simulink model "HMC"  (R2026a)
settings: Solver=ode1  StopTime=inf  FixedStep=0.0001
PreLoadFcn:
  | %load('C:\Users\bme_master\Desktop\mot\mot_6_deneme.mat')
  | 
  | 
  | %load('C:\Users\bme_master\Desktop\mot\PRE_G''s.mat')
PostLoadFcn:
  | , if any(exist('dsrtsu_mdlpostloadfcn', 'file') ~= 0), dsrtsu_mdlpostloadfcn('Execute', bdroot); end,
InitFcn:
  | %motor_control_init_m
  | %clear all
  | %close all
  | %clc
  | b=1e-8
  | StepSize = 1e-4;
  | N=1e-17;
  | 
  | VLV_0 =0;%120; %120
  | VA_0 = 0;%300; %300
  | VRV_0 = 0;%130;
  | VP_0 = 0;%500;
  | VLA_0 = 0;%20;
  | VV_0=5000;
  | VRA_0=0;
  | 
  | 
  | QLV_0 = 0;
  | QLA_0 = 0;
  | QP_0 = 0;
  | 
  | bh = 0;
  | th =0;
  | 
  | X_0 = [VLV_0 VA_0 VV_0 VP_0  VLA_0  VRA_0 VRV_0];
  | 
  | 
  | V0 = 10;
  | 
  | K1=.0004;%0.0001
  | K2=0.0009;%0.0009
  | KA=1;%1
  | C1=0.000000003;%0.0000003
  | lambda=6000;%3000
  | X_00 = [VLV_0 VA_0 VV_0 VRV_0];
  | 
  | r2 = 0.05/2;
  | A2 = pi*r2^2;
  | h2 = 0.63;
  | V2 = A2*h2;
  | 
  | 
  | r3 = 0.05/2;
  | A3 = pi*r3^2;
  | h3 = 0.63;
  | V3 = A3*h3;
  | 
  | 
  | rho = 997;
  | gg = 9.81;
  | %
  | init_min=0;
  | init_max=0;
  | %
  | PWM_Period =  StepSize;
  | PWM_Period_g1 = PWM_Period;
  | PWM_Period_g2 =PWM_Period;
  | PWM_Period_g3 = PWM_Period;
  | PWM_Period_g4 = PWM_Period;
  | PWM_Period_g5 = PWM_Period;
  | ... (+158 lines)
undefined symbols (not defined in the file or in its folder): Continuous, DiscIntNeverNeededParam, Time
libraries: powerlib_meascontrol x19, simulink x15, rti1202lib_adc_class1 x11, cstblocks x10, rti1202lib_dio_class1 x8, dspstat3 x3, rti1202lib_dac_class1 x1, dspswit3 x1, ctrlSharedLib x1, slpidlib x1, dsparch4 x1
(part 4 of 5)

== system HMC/Reference CVSs/eLV/LV_e_min/Real_CLV ==
  note: y = 0,2444x 2 - 30,667x + 2560
      | R² = 1
  Add18 : Sum
  Add19 : Sum
  Constant20 : Constant  Value=25600
  Gain : Gain  Gain=1/100
  Gain2 : Gain  Gain=2.444
  Gain3 : Gain  Gain=- 306.67
  Product15 : Product
  C_LV : Outport
  wires:
  Add19/1 -> Gain/1
  [HR] -> Gain3/1, Product15/2, Product15/1
  Gain2/1 -> Add18/1
  Constant20/1 -> Add19/2
  Product15/1 -> Gain2/1
  Gain3/1 -> Add18/2
  Add18/1 -> Add19/1
  Gain/1 -> C_LV/1

== system HMC/Reference CVSs/eLV/LV_e_min/Subsystem1 ==
  note: y = 0,0446x 2 - 6,3542x + 365,75
      | R² = 1
  Add18 : Sum
  Add19 : Sum
  Constant20 : Constant  Value=365.75
  Gain2 : Gain  Gain=0.0446
  Gain3 : Gain  Gain=- 6.3542
  Product15 : Product
  C_LV : Outport
  wires:
  Add18/1 -> Add19/1
  Gain3/1 -> Add18/2
  Product15/1 -> Gain2/1
  Constant20/1 -> Add19/2
  Gain2/1 -> Add18/1
  [HR] -> Product15/1, Product15/2, Gain3/1
  Add19/1 -> C_LV/1

== system HMC/Reference CVSs/eLV/LV_e_min/Subsystem2 ==
  note: y = 0,0108x 2 - 4,2917x + 398,5
      | R² = 1
  note: y = 0,0011x 2 - 0,4292x + 39,85
      | R² = 1
  note: y = -0,0175x 2 + 5,625x - 264,5
      | R² = 1
  Add18 : Sum
  Add19 : Sum
  Constant20 : Constant  Value=398.5
  Gain : Gain  Gain=1/10000
  Gain2 : Gain  Gain=0.0108
  Gain3 : Gain  Gain=-4.2917
  Product15 : Product
  Scope : Scope
      settings: ActiveDisplayYMinimum=-0.00112  ActiveDisplayYMaximum=0.02012  DataLoggingVariableName=ScopeData2
  B_LV : Outport
  wires:
  Add18/1 -> Add19/1
  Gain3/1 -> Add18/2
  Product15/1 -> Gain2/1
  Constant20/1 -> Add19/2
  Gain2/1 -> Add18/1
  [HR] -> Product15/1, Product15/2, Gain3/1
  Add19/1 -> Gain/1
  Gain/1 -> Scope/1, B_LV/1

== system HMC/Reference CVSs/eLV/LV_e_min/Subsystem5 ==
  note: y = -0,0033x 2 + 0,4333x - 2
      | R² = 1
  Add18 : Sum
  Add19 : Sum
  Constant20 : Constant  Value=-20
  Gain : Gain  Gain=1/10000
  Gain2 : Gain  Gain=-0.0333
  Gain3 : Gain  Gain=4.333
  Product15 : Product
  Scope : Scope
      settings: ActiveDisplayYMinimum=-0.00112  ActiveDisplayYMaximum=0.02012  DataLoggingVariableName=ScopeData2
  B_LV_HF : Outport
  wires:
  Gain/1 -> B_LV_HF/1, Scope/1
  Add19/1 -> Gain/1
  [HR] -> Gain3/1, Product15/2, Product15/1
  Gain2/1 -> Add18/1
  Constant20/1 -> Add19/2
  Product15/1 -> Gain2/1
  Gain3/1 -> Add18/2
  Add18/1 -> Add19/1

== system HMC/Reference CVSs/eLV/LV_e_min/resting ==
  note: y = -4,3333x + 440
  Add19 : Sum
  Constant20 : Constant  Value=440
  Gain : Gain  Gain=1/10000
  Gain3 : Gain  Gain=-4.3333
  Scope : Scope
      settings: ActiveDisplayYMinimum=-0.00112  ActiveDisplayYMaximum=0.02012  DataLoggingVariableName=ScopeData2
  B_LV : Outport
  wires:
  Gain/1 -> B_LV/1, Scope/1
  Add19/1 -> Gain/1
  [insan] -> Gain3/1
  Constant20/1 -> Add19/2
  Gain3/1 -> Add19/1

== system HMC/Reference CVSs/eLV/eLV1/PID ==
  s : Inport
  LTI System : cstblocks/LTI System  sys=tfa  IC=[]
  PID Controller : simulink/Continuous/PID Controller  Controller=PID  Form=Parallel  TimeDomain=Continuous-time  SampleTime=-1  IntegratorMethod=Forward Euler  FilterMethod=Forward Euler  ControllerParametersSource=internal  P=0  I=0.336541519886425  D=0  UseFilter=on  N=100  TunerSelectOption=Transfer Function Based (PID Tuner App)  InitialConditionSource=internal  InitialConditionForIntegrator=0  InitialConditionForFilter=0  DifferentiatorICPrevScaledInput=0  ExternalReset=none  TrackingMode=off  Kt=1  LimitOutput=off  UpperSaturationLimit=inf  LowerSaturationLimit=-inf  LinearizeAsGain=on  AntiWindupMode=none  Kb=1  POutMin=[]  POutMax=[]  IOutMin=[]  IOutMax=[]  DOutMin=[]  DOutMax=[]  NOutMin=[]  NOutMax=[]  SumOutMin=[]  SumOutMax=[]  SaturationOutMin=[]  SaturationOutMax=[]  PParamMin=[]  PParamMax=[]  IParamMin=[]  IParamMax=[]  DParamMin=[]  DParamMax=[]  NParamMin=[]  NParamMax=[]  KbParamMin=[]  KbParamMax=[]  KtParamMin=[]  KtParamMax=[]  KbOutMin=[]  KbOutMax=[]  KtOutMin=[]  KtOutMax=[]  IntegratorOutMin=[]  IntegratorOutMax=[]  FilterOutMin=[]  FilterOutMax=[]  SumI1OutMin=[]  SumI1OutMax=[]  SumI2OutMin=[]  SumI2OutMax=[]  SumI3OutMin=[]  SumI3OutMax=[]  SumI4OutMin=[]  SumI4OutMax=[]  SumDOutMin=[]  SumDOutMax=[]  DifferentiatorOutMin=[]  DifferentiatorOutMax=[]  FilterDiffOutCoefMin=[]  FilterDiffOutCoefMax=[]  ReciprocalOutMin=[]  ReciprocalOutMax=[]  SumDenOutMin=[]  SumDenOutMax=[]  SumNumOutMin=[]  SumNumOutMax=[]  DivideOutMin=[]  DivideOutMax=[]  IntegratorContinuousStateAttributes=''  IntegratorStateMustResolveToSignalObject=off  IntegratorRTWStateStorageClass=Auto  FilterContinuousStateAttributes=''  FilterStateMustResolveToSignalObject=off  FilterRTWStateStorageClass=Auto  ParallelPVariant=InternalParameters  IdealPVariant=Disabled  IVariant=InternalParameters  DVariant=InternalParameters  IntegratorVariant=Continuous  SatVariant=Disabled  AWVariant=Passthrough  PCopyVariant=Disabled  TRVariant=Disabled  FdbkBlocksVariant=Forward  IdealPFdbkVariant=Disabled  SatFdbkVariant=Disabled  DerivativeFilterVariant=ContFilter  NVariant=InternalParameters  NCopyVariant=Disabled  FilterICVariant=InternalICsFilter  IntegratorICVariant=InternalICs  ExternalResetVariant=Disabled  TRSumVariant=Passthrough  SumFdbkVariant=Disabled  SumVariant=Sum_PID
  Sum1 : Sum  Inputs=|+-
  To Workspace : ToWorkspace  VariableName=input  SampleTime=-1
  To Workspace1 : ToWorkspace  VariableName=output  SampleTime=-1
  E : Outport  VectorParamsAs1DForOutWhenUnconnected=off
  wires:
  LTI System/1 -> To Workspace1/1, E/1, Sum1/2
  Sum1/1 -> PID Controller/1
  s/1 -> Sum1/1
  PID Controller/1 -> LTI System/1, To Workspace/1

== system HMC/Reference CVSs/eRV/RV_e_min/c_RV ==
  note: y = 0,0167x 2 - 3,3333x + 290
  Add18 : Sum
  Add19 : Sum
  Constant20 : Constant  Value=290
  Gain2 : Gain  Gain=0.0167
  Gain3 : Gain  Gain=-3.3333
  PID : Subsystem  Commented=on
  Product15 : Product
  Scope : Scope
      settings: ActiveDisplayYMinimum=1.07059  ActiveDisplayYMaximum=1.42514
  Stair Generator : powerlib_meascontrol/Pulse & Signal Generators/Stair Generator  Commented=on  t=[0,50,100,150]  e=[3.25,3.5,3.75,4]  Ts=stepsize
      settings: SourceProductName=Simscape Electrical
  Stair Generator1 : powerlib_meascontrol/Pulse & Signal Generators/Stair Generator  Commented=on  t=[100,200,300,400]  e=[3.25,3.5,3.75,4]  Ts=stepsize
      settings: SourceProductName=Simscape Electrical
  Output : Outport
  wires:
  Stair Generator1/1 -> PID/1(s)
  Gain2/1 -> Add18/1
  Gain3/1 -> Add18/2
  [HR] -> Product15/1, Product15/2, Gain3/1
  Add18/1 -> Add19/1
  Product15/1 -> Gain2/1
  Constant20/1 -> Add19/2
  Add19/1 -> Scope/1, Output/1

== system HMC/Reference CVSs/eRV/RV_e_min/real_c_RV ==
  note: y = - 333,33x + 110000
      | R² = 1
  Add19 : Sum
  Constant20 : Constant  Value=110000
  Gain1 : Gain  Gain=1/1000
  Gain3 : Gain  Gain=-333.33
  PID : Subsystem  Commented=on
  Scope : Scope
      settings: ActiveDisplayYMinimum=1.07059  ActiveDisplayYMaximum=1.42514
  Stair Generator : powerlib_meascontrol/Pulse & Signal Generators/Stair Generator  Commented=on  t=[0,50,100,150]  e=[3.25,3.5,3.75,4]  Ts=stepsize
      settings: SourceProductName=Simscape Electrical
  Stair Generator1 : powerlib_meascontrol/Pulse & Signal Generators/Stair Generator  Commented=on  t=[100,200,300,400]  e=[3.25,3.5,3.75,4]  Ts=stepsize
      settings: SourceProductName=Simscape Electrical
  Output : Outport
  wires:
  Add19/1 -> Gain1/1
  Constant20/1 -> Add19/2
  Gain3/1 -> Add19/1
  [HR] -> Gain3/1
  Stair Generator1/1 -> PID/1(s)
  Gain1/1 -> Output/1, Scope/1

== system HMC/Reference CVSs/eRV/Subsystem2/k_0 ==
  note: y = -0,0042x 2 - 0,0417x + 257,5
      | R² = 1
  In1 : Inport
  Add4 : Sum
  Add5 : Sum
  Constant4 : Constant  Value=257.5
  Gain : Gain  Gain=-0.0041
  Gain1 : Gain  Gain=-0.0417
  Multiply : Gain  Gain=1/1000
  Product8 : Product
  Out1 : Outport
  wires:
  Add4/1 -> Add5/1
  In1/1 -> Gain1/1, Product8/2, Product8/1
  Product8/1 -> Gain/1
  Gain1/1 -> Add4/2
  Gain/1 -> Add4/1
  Constant4/1 -> Add5/2
  Add5/1 -> Multiply/1
  Multiply/1 -> Out1/1

== system HMC/Reference CVSs/eRV/Subsystem2/k_1 ==
  note: y = 0,0158x 2 - 5,0417x + 445,5
      | R² = 1
  In1 : Inport
  Add6 : Sum
  Add7 : Sum
  Constant7 : Constant  Value=445.5
  Gain2 : Gain  Gain=0.0158
  Gain3 : Gain  Gain=-5.0417
  Multiply : Gain  Gain=1/1000
  Product10 : Product
  Out1 : Outport
  wires:
  Constant7/1 -> Add7/2
  Gain2/1 -> Add6/1
  In1/1 -> Gain3/1, Product10/2, Product10/1
  Gain3/1 -> Add6/2
  Add6/1 -> Add7/1
  Product10/1 -> Gain2/1
  Add7/1 -> Multiply/1
  Multiply/1 -> Out1/1

== system HMC/Reference CVSs/eRV/eRV2/PID ==
  s : Inport
  LTI System : cstblocks/LTI System  sys=tfa  IC=[]
  PID Controller : simulink/Continuous/PID Controller  Controller=PID  Form=Parallel  TimeDomain=Continuous-time  SampleTime=-1  IntegratorMethod=Forward Euler  FilterMethod=Forward Euler  ControllerParametersSource=internal  P=0  I=0.336541519886425  D=0  UseFilter=on  N=100  TunerSelectOption=Transfer Function Based (PID Tuner App)  InitialConditionSource=internal  InitialConditionForIntegrator=0  InitialConditionForFilter=0  DifferentiatorICPrevScaledInput=0  ExternalReset=none  TrackingMode=off  Kt=1  LimitOutput=off  UpperSaturationLimit=inf  LowerSaturationLimit=-inf  LinearizeAsGain=on  AntiWindupMode=none  Kb=1  POutMin=[]  POutMax=[]  IOutMin=[]  IOutMax=[]  DOutMin=[]  DOutMax=[]  NOutMin=[]  NOutMax=[]  SumOutMin=[]  SumOutMax=[]  SaturationOutMin=[]  SaturationOutMax=[]  PParamMin=[]  PParamMax=[]  IParamMin=[]  IParamMax=[]  DParamMin=[]  DParamMax=[]  NParamMin=[]  NParamMax=[]  KbParamMin=[]  KbParamMax=[]  KtParamMin=[]  KtParamMax=[]  KbOutMin=[]  KbOutMax=[]  KtOutMin=[]  KtOutMax=[]  IntegratorOutMin=[]  IntegratorOutMax=[]  FilterOutMin=[]  FilterOutMax=[]  SumI1OutMin=[]  SumI1OutMax=[]  SumI2OutMin=[]  SumI2OutMax=[]  SumI3OutMin=[]  SumI3OutMax=[]  SumI4OutMin=[]  SumI4OutMax=[]  SumDOutMin=[]  SumDOutMax=[]  DifferentiatorOutMin=[]  DifferentiatorOutMax=[]  FilterDiffOutCoefMin=[]  FilterDiffOutCoefMax=[]  ReciprocalOutMin=[]  ReciprocalOutMax=[]  SumDenOutMin=[]  SumDenOutMax=[]  SumNumOutMin=[]  SumNumOutMax=[]  DivideOutMin=[]  DivideOutMax=[]  IntegratorContinuousStateAttributes=''  IntegratorStateMustResolveToSignalObject=off  IntegratorRTWStateStorageClass=Auto  FilterContinuousStateAttributes=''  FilterStateMustResolveToSignalObject=off  FilterRTWStateStorageClass=Auto  ParallelPVariant=InternalParameters  IdealPVariant=Disabled  IVariant=InternalParameters  DVariant=InternalParameters  IntegratorVariant=Continuous  SatVariant=Disabled  AWVariant=Passthrough  PCopyVariant=Disabled  TRVariant=Disabled  FdbkBlocksVariant=Forward  IdealPFdbkVariant=Disabled  SatFdbkVariant=Disabled  DerivativeFilterVariant=ContFilter  NVariant=InternalParameters  NCopyVariant=Disabled  FilterICVariant=InternalICsFilter  IntegratorICVariant=InternalICs  ExternalResetVariant=Disabled  TRSumVariant=Passthrough  SumFdbkVariant=Disabled  SumVariant=Sum_PID
  Sum1 : Sum  Inputs=|+-
  To Workspace : ToWorkspace  VariableName=input  SampleTime=-1
  To Workspace1 : ToWorkspace  VariableName=output  SampleTime=-1
  E : Outport  VectorParamsAs1DForOutWhenUnconnected=off
  wires:
  PID Controller/1 -> To Workspace/1, LTI System/1
  s/1 -> Sum1/1
  Sum1/1 -> PID Controller/1
  LTI System/1 -> Sum1/2, E/1, To Workspace1/1

== system HMC/Reference CVSs/eRV/eRVhf/PID ==
  s : Inport
  LTI System : cstblocks/LTI System  sys=tfa  IC=[]
  PID Controller : simulink/Continuous/PID Controller  Controller=PID  Form=Parallel  TimeDomain=Continuous-time  SampleTime=-1  IntegratorMethod=Forward Euler  FilterMethod=Forward Euler  ControllerParametersSource=internal  P=0  I=0.336541519886425  D=0  UseFilter=on  N=100  TunerSelectOption=Transfer Function Based (PID Tuner App)  InitialConditionSource=internal  InitialConditionForIntegrator=0  InitialConditionForFilter=0  DifferentiatorICPrevScaledInput=0  ExternalReset=none  TrackingMode=off  Kt=1  LimitOutput=off  UpperSaturationLimit=inf  LowerSaturationLimit=-inf  LinearizeAsGain=on  AntiWindupMode=none  Kb=1  POutMin=[]  POutMax=[]  IOutMin=[]  IOutMax=[]  DOutMin=[]  DOutMax=[]  NOutMin=[]  NOutMax=[]  SumOutMin=[]  SumOutMax=[]  SaturationOutMin=[]  SaturationOutMax=[]  PParamMin=[]  PParamMax=[]  IParamMin=[]  IParamMax=[]  DParamMin=[]  DParamMax=[]  NParamMin=[]  NParamMax=[]  KbParamMin=[]  KbParamMax=[]  KtParamMin=[]  KtParamMax=[]  KbOutMin=[]  KbOutMax=[]  KtOutMin=[]  KtOutMax=[]  IntegratorOutMin=[]  IntegratorOutMax=[]  FilterOutMin=[]  FilterOutMax=[]  SumI1OutMin=[]  SumI1OutMax=[]  SumI2OutMin=[]  SumI2OutMax=[]  SumI3OutMin=[]  SumI3OutMax=[]  SumI4OutMin=[]  SumI4OutMax=[]  SumDOutMin=[]  SumDOutMax=[]  DifferentiatorOutMin=[]  DifferentiatorOutMax=[]  FilterDiffOutCoefMin=[]  FilterDiffOutCoefMax=[]  ReciprocalOutMin=[]  ReciprocalOutMax=[]  SumDenOutMin=[]  SumDenOutMax=[]  SumNumOutMin=[]  SumNumOutMax=[]  DivideOutMin=[]  DivideOutMax=[]  IntegratorContinuousStateAttributes=''  IntegratorStateMustResolveToSignalObject=off  IntegratorRTWStateStorageClass=Auto  FilterContinuousStateAttributes=''  FilterStateMustResolveToSignalObject=off  FilterRTWStateStorageClass=Auto  ParallelPVariant=InternalParameters  IdealPVariant=Disabled  IVariant=InternalParameters  DVariant=InternalParameters  IntegratorVariant=Continuous  SatVariant=Disabled  AWVariant=Passthrough  PCopyVariant=Disabled  TRVariant=Disabled  FdbkBlocksVariant=Forward  IdealPFdbkVariant=Disabled  SatFdbkVariant=Disabled  DerivativeFilterVariant=ContFilter  NVariant=InternalParameters  NCopyVariant=Disabled  FilterICVariant=InternalICsFilter  IntegratorICVariant=InternalICs  ExternalResetVariant=Disabled  TRSumVariant=Passthrough  SumFdbkVariant=Disabled  SumVariant=Sum_PID
  Sum1 : Sum  Inputs=|+-
  To Workspace : ToWorkspace  VariableName=input  SampleTime=-1
  To Workspace1 : ToWorkspace  VariableName=output  SampleTime=-1
  E : Outport  VectorParamsAs1DForOutWhenUnconnected=off
  wires:
  PID Controller/1 -> To Workspace/1, LTI System/1
  s/1 -> Sum1/1
  Sum1/1 -> PID Controller/1
  LTI System/1 -> Sum1/2, E/1, To Workspace1/1

== system HMC/IBS_LVAD/Subsystem1/Subsystem/Pm1/PID ==
  s : Inport
  LTI System : cstblocks/LTI System  sys=tfa  IC=[]
  PID Controller : simulink/Continuous/PID Controller  Controller=PID  Form=Parallel  TimeDomain=Continuous-time  SampleTime=-1  IntegratorMethod=Forward Euler  FilterMethod=Forward Euler  ControllerParametersSource=internal  P=0  I=0.336541519886425  D=0  UseFilter=on  N=100  TunerSelectOption=Transfer Function Based (PID Tuner App)  InitialConditionSource=internal  InitialConditionForIntegrator=0  InitialConditionForFilter=0  DifferentiatorICPrevScaledInput=0  ExternalReset=none  TrackingMode=off  Kt=1  LimitOutput=off  UpperSaturationLimit=inf  LowerSaturationLimit=-inf  LinearizeAsGain=on  AntiWindupMode=none  Kb=1  POutMin=[]  POutMax=[]  IOutMin=[]  IOutMax=[]  DOutMin=[]  DOutMax=[]  NOutMin=[]  NOutMax=[]  SumOutMin=[]  SumOutMax=[]  SaturationOutMin=[]  SaturationOutMax=[]  PParamMin=[]  PParamMax=[]  IParamMin=[]  IParamMax=[]  DParamMin=[]  DParamMax=[]  NParamMin=[]  NParamMax=[]  KbParamMin=[]  KbParamMax=[]  KtParamMin=[]  KtParamMax=[]  KbOutMin=[]  KbOutMax=[]  KtOutMin=[]  KtOutMax=[]  IntegratorOutMin=[]  IntegratorOutMax=[]  FilterOutMin=[]  FilterOutMax=[]  SumI1OutMin=[]  SumI1OutMax=[]  SumI2OutMin=[]  SumI2OutMax=[]  SumI3OutMin=[]  SumI3OutMax=[]  SumI4OutMin=[]  SumI4OutMax=[]  SumDOutMin=[]  SumDOutMax=[]  DifferentiatorOutMin=[]  DifferentiatorOutMax=[]  FilterDiffOutCoefMin=[]  FilterDiffOutCoefMax=[]  ReciprocalOutMin=[]  ReciprocalOutMax=[]  SumDenOutMin=[]  SumDenOutMax=[]  SumNumOutMin=[]  SumNumOutMax=[]  DivideOutMin=[]  DivideOutMax=[]  IntegratorContinuousStateAttributes=''  IntegratorStateMustResolveToSignalObject=off  IntegratorRTWStateStorageClass=Auto  FilterContinuousStateAttributes=''  FilterStateMustResolveToSignalObject=off  FilterRTWStateStorageClass=Auto  ParallelPVariant=InternalParameters  IdealPVariant=Disabled  IVariant=InternalParameters  DVariant=InternalParameters  IntegratorVariant=Continuous  SatVariant=Disabled  AWVariant=Passthrough  PCopyVariant=Disabled  TRVariant=Disabled  FdbkBlocksVariant=Forward  IdealPFdbkVariant=Disabled  SatFdbkVariant=Disabled  DerivativeFilterVariant=ContFilter  NVariant=InternalParameters  NCopyVariant=Disabled  FilterICVariant=InternalICsFilter  IntegratorICVariant=InternalICs  ExternalResetVariant=Disabled  TRSumVariant=Passthrough  SumFdbkVariant=Disabled  SumVariant=Sum_PID
  Sum1 : Sum  Inputs=|+-
  To Workspace : ToWorkspace  VariableName=input  SampleTime=-1
  To Workspace1 : ToWorkspace  VariableName=output  SampleTime=-1
  E : Outport  VectorParamsAs1DForOutWhenUnconnected=off
  wires:
  LTI System/1 -> To Workspace1/1, E/1, Sum1/2
  Sum1/1 -> PID Controller/1
  s/1 -> Sum1/1
  PID Controller/1 -> LTI System/1, To Workspace/1

== system HMC/IBS_LVAD/Subsystem1/Subsystem/Pressures Flows and Volumes1/Exercise ==
  note: y = 0,0167x 2 + 0,6667x + 180
  note: y = -0,0033x 2 + 0,8667x - 16
  HR1 : Inport
  Enable : EnablePort
  Add{4..5,18..19} (4 alike) : Sum
  Constant20 : Constant  Value=0.5621
  Constant4 : Constant  Value=-16
  Gain2 : Gain  Gain=0.000003
  Gain3 : Gain  Gain=-0.0008
  Gain5 : Gain  Gain=1/10000
  Gain6 : Gain  Gain=-0.0033
  Gain7 : Gain  Gain=0.8667
  Mux : Mux  Inputs=2
  Product15 : Product
  Product3 : Product
  Output : Outport
  wires:
  Add19/1 -> Mux/2  "eA"
  Product15/1 -> Gain2/1
  Constant20/1 -> Add19/2
  Add18/1 -> Add19/1
  Gain3/1 -> Add18/2
  Gain2/1 -> Add18/1
  HR1/1 -> Product15/1, Product15/2, Gain3/1, Gain7/1, Product3/2, Product3/1
  Mux/1 -> Output/1
  Constant4/1 -> Add5/2
  Add4/1 -> Add5/1
  Gain6/1 -> Add4/1
  Add5/1 -> Gain5/1
  Gain5/1 -> Mux/1
  Product3/1 -> Gain6/1
  Gain7/1 -> Add4/2

== system HMC/IBS_LVAD/Subsystem1/Subsystem/Pressures Flows and Volumes1/Exercise2 ==
  HR : Inport
  Enable : EnablePort
  Add{5..8,11..12,18..19} (8 alike) : Sum
  Constant20 : Constant  Value=-3650
  Constant4 : Constant  Value=12500
  Constant5 : Constant  Value=-18.5
  Constant7 : Constant  Value=600.5
  Gain : Gain  Gain=1/1000
  Gain10 : Gain  Gain=3041.7
  Gain11 : Gain  Gain=1/100
  Gain12 : Gain  Gain=0.0058
  Gain13 : Gain  Gain=1.4583
  Gain16 : Gain
  Gain17 : Gain  Gain=0.0742
  Gain18 : Gain  Gain=-10.958
  Gain2 : Gain  Gain=0.25
  Gain3 : Gain  Gain=1212.5
  Gain8 : Gain  Gain=1/1000
  Gain9 : Gain  Gain=4.1667
  Mux : Mux
  Product{2..3,5,15} (4 alike) : Product
  Scope : Scope
      settings: ActiveDisplayYMinimum=60  ActiveDisplayYMaximum=80  DataLoggingVariableName=ScopeData9
  Output : Outport
  wires:
  Gain9/1 -> Add5/1
  Product2/1 -> Gain9/1
  Add5/1 -> Add6/1
  Gain8/1 -> Mux/3
  Gain10/1 -> Add5/2
  Constant4/1 -> Add6/2
  Add6/1 -> Gain8/1
  Add18/1 -> Add19/1
  Add19/1 -> Gain/1
  Gain3/1 -> Add18/2
  Product15/1 -> Gain2/1
  Constant20/1 -> Add19/2
  Gain/1 -> Scope/1, Mux/1
  Gain2/1 -> Add18/1
  Mux/1 -> Output/1
  Gain12/1 -> Add7/1
  Add7/1 -> Add8/1
  Constant5/1 -> Add8/2
  Product3/1 -> Gain12/1
  Add8/1 -> Gain11/1
  Gain11/1 -> Mux/2
  Gain13/1 -> Add7/2
  Product5/1 -> Gain17/1
  Add11/1 -> Add12/1
  Constant7/1 -> Add12/2
  Add12/1 -> Gain16/1
  HR/1 -> Gain3/1, Product15/2, Product15/1, Gain10/1, Product2/2, Product2/1, Product5/1, Product5/2, Gain18/1, Gain13/1, Product3/2, Product3/1
  Gain17/1 -> Add11/1
  Gain16/1 -> Mux/4
  Gain18/1 -> Add11/2

== system HMC/IBS_LVAD/Subsystem1/Subsystem/Pressures Flows and Volumes1/Rest ==
  note: eC
  note: y = -0,0033x 2 + 0,8667x - 16
  note: eRA
  note: eLA
  note: eP
  note: y = 0,5x + 40
  note: eV
  HR : Inport
  Input : Inport  Port=2
  Enable : EnablePort
  Add18 : Sum
  Add19 : Sum
  Add7 : Sum
  Constant20 : Constant  Value=-16
  Constant4 : Constant  Value=40
  Gain1 : Gain  Gain=1/10000
  Gain12 : Gain  Gain=1/100
  Gain13 : Gain  Gain=0.5
  Gain2 : Gain  Gain=-0.0033
  Gain3 : Gain  Gain=0.8667
  Mux : Mux  Inputs=2
  Product15 : Product
  Output : Outport
  wires:
  Gain3/1 -> Add18/2
  Product15/1 -> Gain2/1
  Add19/1 -> Gain1/1
  Constant20/1 -> Add19/2
  Gain2/1 -> Add18/1
  Add18/1 -> Add19/1
  Gain1/1 -> Mux/1
  Mux/1 -> Output/1
  HR/1 -> Gain3/1, Product15/2, Product15/1
  Add7/1 -> Gain12/1
  Constant4/1 -> Add7/2
  Gain13/1 -> Add7/1
  Gain12/1 -> Mux/2  "eA"
  Input/1 -> Gain13/1

== system HMC/IBS_LVAD/Subsystem1/Subsystem/Pressures Flows and Volumes1/Rest1 ==
  HR : Inport
  Input : Inport  Port=2
  Enable : EnablePort
  Add{5..10,18..19} (8 alike) : Sum
  Constant20 : Constant  Value=-3650
  Constant4 : Constant  Value=12500
  Constant5 : Constant  Value=-45
  Constant6 : Constant  Value=600.5
  Gain : Gain  Gain=1/1000
  Gain10 : Gain  Gain=3041.7
  Gain11 : Gain  Gain=1/100
  Gain12 : Gain  Gain=-0.0167
  Gain13 : Gain  Gain=3.25
  Gain14 : Gain
  Gain15 : Gain  Gain=0.0742
  Gain16 : Gain  Gain=-10.958
  Gain2 : Gain  Gain=0.25
  Gain3 : Gain  Gain=1212.5
  Gain8 : Gain  Gain=1/1000
  Gain9 : Gain  Gain=4.1667
  Mux : Mux
  Product{2..4,15} (4 alike) : Product
  Scope : Scope
      settings: ActiveDisplayYMinimum=60  ActiveDisplayYMaximum=80  DataLoggingVariableName=ScopeData9
  Output : Outport
  wires:
  Mux/1 -> Output/1
  Gain2/1 -> Add18/1
  Gain/1 -> Mux/1, Scope/1
  Constant20/1 -> Add19/2
  Product15/1 -> Gain2/1
  Gain3/1 -> Add18/2
  Add19/1 -> Gain/1
  Add18/1 -> Add19/1
  Add6/1 -> Gain8/1
  Constant4/1 -> Add6/2
  Gain10/1 -> Add5/2
  Gain8/1 -> Mux/3
  Add5/1 -> Add6/1
  Product2/1 -> Gain9/1
  Gain9/1 -> Add5/1
  Gain13/1 -> Add7/2
  Add7/1 -> Add8/1
  Product3/1 -> Gain12/1
  Constant5/1 -> Add8/2
  Add8/1 -> Gain11/1
  Gain12/1 -> Add7/1
  Input/1 -> Product3/1, Product3/2, Gain13/1
  Gain11/1 -> Mux/2
  Product4/1 -> Gain15/1
  Add9/1 -> Add10/1
  Constant6/1 -> Add10/2
  Add10/1 -> Gain14/1
  HR/1 -> Product4/1, Product4/2, Gain16/1, Product2/1, Product2/2, Gain10/1, Product15/1, Product15/2, Gain3/1
  Gain15/1 -> Add9/1
  Gain14/1 -> Mux/4
  Gain16/1 -> Add9/2

== system HMC/IBS_LVAD/Subsystem1/Subsystem/Pressures Flows and Volumes1/Subsystem ==
  In1 : Inport
  Add7 : Sum
  Add8 : Sum
  Constant5 : Constant  Value=4.6
  Gain11 : Gain  Gain=1/100
  Gain12 : Gain  Gain=0.0003
  Gain13 : Gain  Gain=-0.0367
  Product4 : Product
  Out1 : Outport
  wires:
  Gain11/1 -> Out1/1
  In1/1 -> Gain13/1, Product4/2, Product4/1
  Add7/1 -> Add8/1
  Gain12/1 -> Add7/1
  Add8/1 -> Gain11/1
  Constant5/1 -> Add8/2
  Product4/1 -> Gain12/1
  Gain13/1 -> Add7/2

== system HMC/IBS_LVAD/Subsystem1/Subsystem/Pressures Flows and Volumes1/Subsystem13 ==
  note: y = 0,1944x 2 - 28,333x + 1100
  Add18 : Sum
  Add19 : Sum
  Constant20 : Constant  Value=1100
  Display : Display
  Gain : Gain  Gain=1/10
  Gain2 : Gain  Gain=0.1944
  Gain3 : Gain  Gain=-28.333
  Product15 : Product
  Scope : Scope
      settings: ActiveDisplayYMinimum=8.99968  ActiveDisplayYMaximum=10.99968  DataLoggingVariableName=ScopeData2
  V0 : Outport
  wires:
  Add19/1 -> Gain/1
  Add18/1 -> Add19/1
  Gain3/1 -> Add18/2
  Product15/1 -> Gain2/1
  Constant20/1 -> Add19/2
  Gain2/1 -> Add18/1
  [HR] -> Product15/1, Product15/2, Gain3/1
  Gain/1 -> Scope/1, Display/1, V0/1

== system HMC/IBS_LVAD/Subsystem1/Subsystem/eLV1/LV_e_min ==
  VLV : Inport
  Add : Sum  Inputs=+-
  Add1 : Sum  Inputs=+-
  Add2 : Sum
  Constant : Constant  Value=.00185
  Constant9 : Constant
  Display : Display
  Display1 : Display
  Exp : Math  SignedPower=on
  Product : Product
  Product1 : Product
  Subsystem1 : Subsystem
  Subsystem2 : Subsystem
  Switch2 : Switch  Criteria=u2 > Threshold  SaturateOnIntegerOverflow=off  InputSameDT=off
  a_LV_Cons : Constant  Value=0.4641
  d_LV_Cons : Constant  Value=0.1235
  resting : Subsystem
  eLV_min_O : Outport
  wires:
  Add/1 -> Product1/2
  Product1/1 -> Exp/1
  Exp/1 -> Add1/1
  d_LV_Cons/1 -> Add2/2
  Product/1 -> Add2/1
  Add1/1 -> Product/2
  Constant9/1 -> Add1/2
  VLV/1 -> Add/1
  Add2/1 -> eLV_min_O/1
  a_LV_Cons/1 -> Product/1
  [Exercise_REF] -> Switch2/2
  resting/1(B_LV) -> Switch2/3
  Subsystem2/1(B_LV) -> Switch2/1
  Constant/1 -> Product1/1, Display/1
  Subsystem1/1(C_LV) -> Add/2, Display1/1

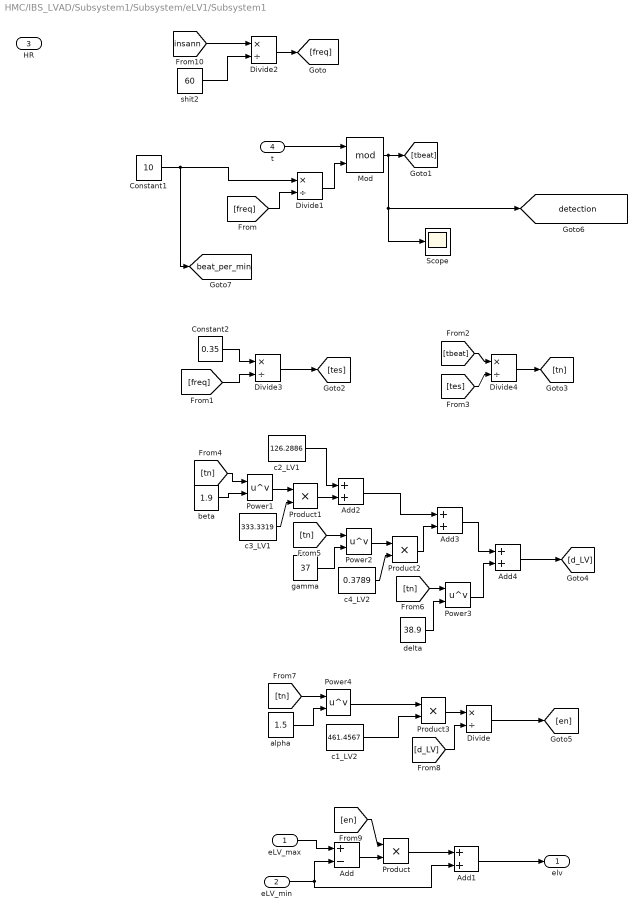
== system HMC/IBS_LVAD/Subsystem1/Subsystem/eLV1/Subsystem1 ==
  eLV_max : Inport
  eLV_min : Inport  Port=2
  HR : Inport  Port=3
  t : Inport  Port=4
  Add : Sum  Inputs=+-
  Add{1..4} (4 alike) : Sum
  Constant1 : Constant  Value=10
  Constant2 : Constant  Value=0.35
  Divide{,1..4} (5 alike) : Product  Inputs=*/  RndMeth=Zero  SaturateOnIntegerOverflow=on
  Mod : Math  Operator=mod  SignedPower=on
  Power{1..4} (4 alike) : Math  Operator=pow  SignedPower=on
  Product{,1..3} (4 alike) : Product
  Scope : Scope
      settings: ActiveDisplayYMinimum=-1.24999  ActiveDisplayYMaximum=11.24989  DataLoggingVariableName=ScopeData4
  alpha : Constant  Value=1.5
  beta : Constant  Value=1.9
  c1_LV2 : Constant  Value=461.4567
  c2_LV1 : Constant  Value=126.2886
  c3_LV1 : Constant  Value=333.3319
  c4_LV2 : Constant  Value=0.3789
  delta : Constant  Value=38.9
  gamma : Constant  Value=37
  "shit2 " : Constant  Value=60
  elv : Outport
  tag scope: beat_per_min=global, detection=global
  wires:
  Product/1 -> Add1/1
  Add/1 -> Product/2
  Add1/1 -> elv/1
  eLV_min/1 -> Add/2, Add1/2
  eLV_max/1 -> Add/1
  "shit2 "/1 -> Divide2/2
  Divide2/1 -> [freq]
  [freq] -> Divide1/2
  Constant1/1 -> [beat_per_min], Divide1/1
  Constant2/1 -> Divide3/1
  [freq] -> Divide3/2
  Divide3/1 -> [tes]
  [tbeat] -> Divide4/1
  [tes] -> Divide4/2
  Divide4/1 -> [tn]
  c2_LV1/1 -> Add2/1
  [tn] -> Power1/1
  beta/1 -> Power1/2
  Power1/1 -> Product1/1
  c3_LV1/1 -> Product1/2
  Product1/1 -> Add2/2
  Add2/1 -> Add3/1
  [tn] -> Power2/1
  gamma/1 -> Power2/2
  Power2/1 -> Product2/1
  c4_LV2/1 -> Product2/2
  Product2/1 -> Add3/2
  [tn] -> Power3/1
  delta/1 -> Power3/2
  Add3/1 -> Add4/1
  Power3/1 -> Add4/2
  Add4/1 -> [d_LV]
  [tn] -> Power4/1
  alpha/1 -> Power4/2
  Power4/1 -> Product3/1
  c1_LV2/1 -> Product3/2
  Product3/1 -> Divide/1
  Divide/1 -> [en]
  [d_LV] -> Divide/2
  [en] -> Product/1
  t/1 -> Mod/1
  Divide1/1 -> Mod/2
  [insann] -> Divide2/1
  Mod/1 -> Scope/1, [detection], [tbeat]

== system HMC/IBS_LVAD/Subsystem1/Subsystem/eLV1/eLV1 ==
  note: y = 0,0027x 2 - 0,0767x + 24,76
  Add18 : Sum
  Add19 : Sum
  Constant20 : Constant  Value=24.76
  Gain1 : Gain  Gain=1/10
  Gain2 : Gain  Gain=0.0027
  Gain3 : Gain  Gain=-0.0767
  PID : Subsystem  Commented=on
  Product15 : Product
  Scope : Scope
      settings: ActiveDisplayYMinimum=2.20237  ActiveDisplayYMaximum=2.60692
  Stair Generator : powerlib_meascontrol/Pulse & Signal Generators/Stair Generator  Commented=on  t=[0,50,100,150]  e=[3.25,3.5,3.75,4]  Ts=stepsize
      settings: SourceProductName=Simscape Electrical
  Stair Generator1 : powerlib_meascontrol/Pulse & Signal Generators/Stair Generator  Commented=on  t=[100,200,300,400]  e=[3.25,3.5,3.75,4]  Ts=stepsize
      settings: SourceProductName=Simscape Electrical
  Output : Outport
  wires:
  Stair Generator1/1 -> PID/1(s)
  Add19/1 -> Gain1/1
  Gain2/1 -> Add18/1
  Gain3/1 -> Add18/2
  [HR] -> Product15/1, Product15/2, Gain3/1
  Add18/1 -> Add19/1
  Product15/1 -> Gain2/1
  Constant20/1 -> Add19/2
  Gain1/1 -> Scope/1, Output/1

== system HMC/IBS_LVAD/Subsystem1/Subsystem/eRV1/RV_e_min ==
  VRV : Inport
  Add3 : Sum  Inputs=+-
  Add4 : Sum
  Constant13 : Constant
  Display1 : Display
  Exp1 : Math  SignedPower=on
  Product2 : Product
  Product3 : Product
  a_RV_Cons : Constant  Value=0.03752
  b_RV_Cons : Constant  Value=0.03776
  c_RV : Subsystem
  eRV_min_O : Outport
  wires:
  Constant13/1 -> Add4/2
  Product2/1 -> Exp1/1
  Add3/1 -> Product2/1
  VRV/1 -> Add3/1
  Exp1/1 -> Add4/1
  Add4/1 -> Product3/2
  c_RV/1(Output) -> Display1/1, Add3/2
  a_RV_Cons/1 -> Product3/1
  b_RV_Cons/1 -> Product2/2
  Product3/1 -> eRV_min_O/1

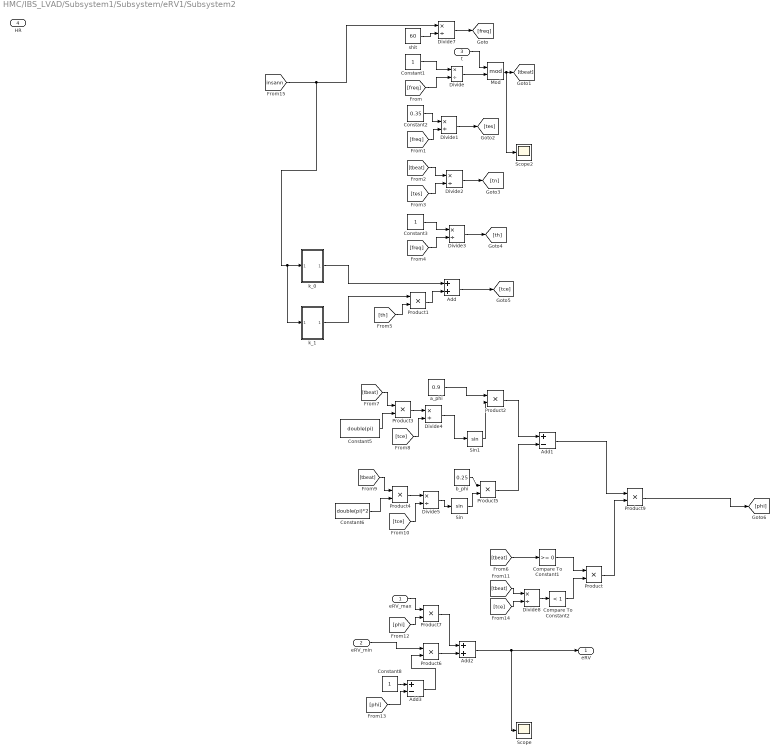
== system HMC/IBS_LVAD/Subsystem1/Subsystem/eRV1/Subsystem2 ==
  eRV_max : Inport
  eRV_min : Inport  Port=2
  t : Inport  Port=3
  HR : Inport  Port=4
  Add : Sum
  Add1 : Sum  Inputs=+-
  Add2 : Sum
  Add3 : Sum  Inputs=+-
  Compare To Constant1 : simulink/Logic and Bit Operations/Compare To Constant  relop=>=  const=0  OutDataTypeStr=boolean
  Compare To Constant2 : simulink/Logic and Bit Operations/Compare To Constant  relop=<  const=1  OutDataTypeStr=boolean
  Constant1 : Constant
  Constant2 : Constant  Value=0.35
  Constant3 : Constant
  Constant5 : Constant  Value=double(pi)
  Constant6 : Constant  Value=double(pi)*2
  Constant8 : Constant
  Divide{,1..5,7..8} (8 alike) : Product  Inputs=*/  RndMeth=Zero  SaturateOnIntegerOverflow=on
  Mod : Math  Operator=mod  SignedPower=on
  Product{,1..7,9} (9 alike) : Product
  Scope : Scope
      settings: ActiveDisplayYMinimum=-0.03117  ActiveDisplayYMaximum=2.17237  DataLoggingVariableName=ScopeData3
  Scope2 : Scope
      settings: ActiveDisplayYMinimum=-0.09374  ActiveDisplayYMaximum=0.84364  DataLoggingVariableName=ScopeData6
  Sin : Trigonometry
  Sin1 : Trigonometry
  a_phi : Constant  Value=0.9
  b_phi : Constant  Value=0.25
  k_0 : Subsystem
  k_1 : Subsystem
  shit : Constant  Value=60
  eRV : Outport
  wires:
  shit/1 -> Divide7/2
  Divide7/1 -> [freq]
  Constant1/1 -> Divide/1
  [freq] -> Divide/2
  Mod/1 -> Scope2/1, [tbeat]
  Constant2/1 -> Divide1/1
  [freq] -> Divide1/2
  Divide1/1 -> [tes]
  [tbeat] -> Divide2/1
  [tes] -> Divide2/2
  Divide2/1 -> [tn]
  Constant3/1 -> Divide3/1
  [freq] -> Divide3/2
  Divide3/1 -> [th]
  [th] -> Product1/2
  Add/1 -> [tce]
  Product1/1 -> Add/2
  [tbeat] -> Compare To Constant1/1
  a_phi/1 -> Product2/1
  [tbeat] -> Product3/1
  Constant5/1 -> Product3/2
  Product3/1 -> Divide4/1
  [tce] -> Divide4/2
  Product2/1 -> Add1/1
  Divide5/1 -> Sin/1
  Constant6/1 -> Product4/2
  [tce] -> Divide5/2
  [tbeat] -> Product4/1
  Product4/1 -> Divide5/1
  Sin/1 -> Product5/2
  b_phi/1 -> Product5/1
  Product5/1 -> Add1/2
  Add1/1 -> Product9/1
  Product9/1 -> [phi]
  eRV_min/1 -> Product6/1
  Product6/1 -> Add2/2
  eRV_max/1 -> Product7/1
  [phi] -> Product7/2
  Product7/1 -> Add2/1
  Add2/1 -> Scope/1, eRV/1
  Constant8/1 -> Add3/1
  [phi] -> Add3/2
  Add3/1 -> Product6/2
  Divide/1 -> Mod/2
  t/1 -> Mod/1
  [tbeat] -> Divide8/1
  [tce] -> Divide8/2
  Divide8/1 -> Compare To Constant2/1
  Compare To Constant1/1 -> Product/1
  Compare To Constant2/1 -> Product/2
  Product/1 -> Product9/2
  Divide4/1 -> Sin1/1
  Sin1/1 -> Product2/2
  k_1/1(Out1) -> Product1/1
  k_0/1(Out1) -> Add/1
  [insann] -> k_1/1(In1), k_0/1(In1), Divide7/1

== system HMC/IBS_LVAD/Subsystem1/Subsystem/eRV1/eRV2 ==
  note: y = 0,005x 2 + 0,25x + 17
  Add18 : Sum
  Add19 : Sum
  Constant20 : Constant  Value=17
  Gain1 : Gain  Gain=1/100
  Gain2 : Gain  Gain=0.005
  Gain3 : Gain  Gain=0.25
  PID : Subsystem  Commented=on
  Product15 : Product
  Scope : Scope
      settings: ActiveDisplayYMinimum=1.07059  ActiveDisplayYMaximum=1.42514
  Stair Generator : powerlib_meascontrol/Pulse & Signal Generators/Stair Generator  Commented=on  t=[0,50,100,150]  e=[3.25,3.5,3.75,4]  Ts=stepsize
      settings: SourceProductName=Simscape Electrical
  Stair Generator1 : powerlib_meascontrol/Pulse & Signal Generators/Stair Generator  Commented=on  t=[100,200,300,400]  e=[3.25,3.5,3.75,4]  Ts=stepsize
      settings: SourceProductName=Simscape Electrical
  Output : Outport
  wires:
  Gain1/1 -> Output/1, Scope/1
  Constant20/1 -> Add19/2
  Product15/1 -> Gain2/1
  Add18/1 -> Add19/1
  [HR] -> Gain3/1, Product15/2, Product15/1
  Gain3/1 -> Add18/2
  Gain2/1 -> Add18/1
  Add19/1 -> Gain1/1
  Stair Generator1/1 -> PID/1(s)

== system HMC/RTI Data/RTI Data Store/RTI Data Store/RTI Data Store/RTI Data Store ==

== system HMC/Reference CVSs/Pressures Flows and Volumes/Subsystem5/VolumesForVAD/Subsystem13 ==
  note: y = 0,1944x 2 - 28,333x + 1100
  Add{1..2,18..19} (4 alike) : Sum
  Constant1 : Constant  Value=2750
  Constant20 : Constant  Value=1100
  Display : Display
  Gain : Gain  Gain=1/10
  Gain1 : Gain  Gain=1/1000
  Gain2 : Gain  Gain=0.1944
  Gain3 : Gain  Gain=-28.333
  Gain4 : Gain  Gain=-0.4167
  Gain5 : Gain  Gain=145.83
  Product1 : Product
  Product15 : Product
  Scope : Scope
      settings: ActiveDisplayYMinimum=8.99968  ActiveDisplayYMaximum=10.99968  DataLoggingVariableName=ScopeData2
  Scope1 : Scope
      settings: ActiveDisplayYMinimum=8.99968  ActiveDisplayYMaximum=10.99968
  Switch : Switch  Criteria=u2 > Threshold  SaturateOnIntegerOverflow=off  InputSameDT=off
  V0 : Outport
  wires:
  Add19/1 -> Gain/1
  Add18/1 -> Add19/1
  Gain3/1 -> Add18/2
  Product15/1 -> Gain2/1
  Constant20/1 -> Add19/2
  Gain2/1 -> Add18/1
  [HR] -> Product15/1, Product15/2, Gain3/1
  Gain/1 -> Switch/1, Scope/1
  Gain1/1 -> Switch/3, Scope1/1
  [HR] -> Gain5/1, Product1/2, Product1/1
  Gain4/1 -> Add1/1
  Constant1/1 -> Add2/2
  Product1/1 -> Gain4/1
  Gain5/1 -> Add1/2
  Add1/1 -> Add2/1
  Add2/1 -> Gain1/1
  [Heart_Failure_On_Off] -> Switch/2
  Switch/1 -> Display/1, V0/1

== system HMC/Reference CVSs/Pressures Flows and Volumes/Subsystem5/VolumesForVAD/Subsystem15 ==
  note: y = -0,0278x 2 + 5,8333x - 150
  Add18 : Sum
  Add19 : Sum
  Constant20 : Constant  Value=-150
  Gain2 : Gain  Gain=-0.0278
  Gain3 : Gain  Gain=5.8333
  Multiply : Gain  Gain=1/100
  Product15 : Product
  Scope : Scope
      settings: ActiveDisplayYMinimum=0.50527  ActiveDisplayYMaximum=0.53249  DataLoggingVariableName=ScopeData2
  eAO : Outport
  wires:
  Add19/1 -> Multiply/1
  Add18/1 -> Add19/1
  Gain3/1 -> Add18/2
  Product15/1 -> Gain2/1
  Constant20/1 -> Add19/2
  Gain2/1 -> Add18/1
  [HR] -> Product15/1, Product15/2, Gain3/1
  Multiply/1 -> eAO/1, Scope/1

== system HMC/Reference CVSs/Pressures Flows and Volumes/Subsystem5/VolumesForVAD/Subsystem17 ==
  note: y = -0,0033x 2 + 0,8667x - 16
  Add18 : Sum
  Add19 : Sum
  Constant20 : Constant  Value=-16
  Gain1 : Gain  Gain=1/10000
  Gain2 : Gain  Gain=-0.0033
  Gain3 : Gain  Gain=0.8667
  Product15 : Product
  Scope : Scope
      settings: ActiveDisplayYMinimum=0.00132  ActiveDisplayYMaximum=0.00154  DataLoggingVariableName=ScopeData2
  eV : Outport
  wires:
  Gain1/1 -> eV/1, Scope/1
  Add19/1 -> Gain1/1
  [HR] -> Gain3/1, Product15/2, Product15/1
  Gain2/1 -> Add18/1
  Constant20/1 -> Add19/2
  Product15/1 -> Gain2/1
  Gain3/1 -> Add18/2
  Add18/1 -> Add19/1

== system HMC/Reference CVSs/Pressures Flows and Volumes/Subsystem5/VolumesForVAD/Subsystem18 ==
  note: y = 0,0167x 2 - 5,8333x + 1290
      | R² = 1
  Add19 : Sum
  Constant20 : Constant  Value=1150
  Gain3 : Gain  Gain=-2.5
  Scope : Scope
      settings: ActiveDisplayYMinimum=900  ActiveDisplayYMaximum=1100  DataLoggingVariableName=ScopeData2
  gRA : Outport
  wires:
  Constant20/1 -> Add19/2
  [HR] -> Gain3/1
  Add19/1 -> Scope/1, gRA/1
  Gain3/1 -> Add19/1

== system HMC/Reference CVSs/Pressures Flows and Volumes/Subsystem5/VolumesForVAD/Subsystem19 ==
  note: y = - 5x + 1300R² = 1
  note: y = 0,0167x 2 - 5,8333x + 1290
      | R² = 1
  Add19 : Sum
  Constant20 : Constant  Value=1300
  Gain3 : Gain  Gain=-5
  Scope : Scope
      settings: ActiveDisplayYMinimum=900  ActiveDisplayYMaximum=1100  DataLoggingVariableName=ScopeData2
  gLA : Outport
  wires:
  Add19/1 -> gLA/1, Scope/1
  [HR] -> Gain3/1
  Constant20/1 -> Add19/2
  Gain3/1 -> Add19/1

== system HMC/Reference CVSs/Pressures Flows and Volumes/Subsystem5/VolumesForVAD/Subsystem20 ==
  note: y = 0,0058x 2 + 1,4583x - 18,5
  Add18 : Sum
  Add19 : Sum
  Constant20 : Constant  Value=-18.5
  Gain1 : Gain  Gain=1/100
  Gain2 : Gain  Gain=0.0058
  Gain3 : Gain  Gain=1.4583
  Product15 : Product
  Scope : Scope
      settings: ActiveDisplayYMinimum=0.88246  ActiveDisplayYMaximum=1.08246  DataLoggingVariableName=ScopeData2
  gAO : Outport
  wires:
  Gain1/1 -> gAO/1, Scope/1
  Add19/1 -> Gain1/1
  [HR] -> Gain3/1, Product15/2, Product15/1
  Gain2/1 -> Add18/1
  Constant20/1 -> Add19/2
  Product15/1 -> Gain2/1
  Gain3/1 -> Add18/2
  Add18/1 -> Add19/1

== system HMC/Reference CVSs/Pressures Flows and Volumes/Subsystem5/VolumesForVAD/Subsystem21 ==
  note: y = 0,0742x 2 - 10,958x + 600,5
  Add18 : Sum
  Add19 : Sum
  Constant20 : Constant  Value=600.5
  Gain : Gain
  Gain2 : Gain  Gain=0.0742
  Gain3 : Gain  Gain=-10.958
  Product15 : Product
  Scope : Scope
      settings: ActiveDisplayYMinimum=109.99968  ActiveDisplayYMaximum=309.99968  DataLoggingVariableName=ScopeData2
  gRV : Outport
  wires:
  Gain/1 -> Scope/1, gRV/1
  Add18/1 -> Add19/1
  Gain3/1 -> Add18/2
  Product15/1 -> Gain2/1
  Constant20/1 -> Add19/2
  Gain2/1 -> Add18/1
  [HR] -> Product15/1, Product15/2, Gain3/1
  Add19/1 -> Gain/1

== system HMC/Reference CVSs/Pressures Flows and Volumes/Subsystem5/VolumesForVAD/Subsystem23 ==
  note: y = 0,1417x 2 - 24,583x + 2165
  Add18 : Sum
  Add19 : Sum
  Constant20 : Constant  Value=2165
  Gain : Gain  Gain=1/10000
  Gain2 : Gain  Gain=0.1417
  Gain3 : Gain  Gain=-24.583
  Product15 : Product
  Scope : Scope
      settings: ActiveDisplayYMinimum=0.01994  ActiveDisplayYMaximum=0.21994  DataLoggingVariableName=ScopeData2
  eP : Outport
  wires:
  Gain/1 -> Scope/1, eP/1
  Add18/1 -> Add19/1
  Gain3/1 -> Add18/2
  Product15/1 -> Gain2/1
  Constant20/1 -> Add19/2
  Gain2/1 -> Add18/1
  [HR] -> Product15/1, Product15/2, Gain3/1
  Add19/1 -> Gain/1

== system HMC/Reference CVSs/Pressures Flows and Volumes/Subsystem5/VolumesForVAD/Subsystem24 ==
  note: y = -2E-06x 2 + 0,0011x + 0,044
      | R² = 1
  note: y = -0,0069x2 + 1,2813x + 30,375R² = 1
  Add18 : Sum
  Add19 : Sum
  Constant20 : Constant  Value=30.375
  Gain : Gain  Gain=1/1000
  Gain2 : Gain  Gain=-0.0069
  Gain3 : Gain  Gain=1.2813
  Product15 : Product
  Scope : Scope
      settings: ActiveDisplayYMinimum=0.07241  ActiveDisplayYMaximum=0.09241  DataLoggingVariableName=ScopeData2
  eLA : Outport
  wires:
  Gain/1 -> Scope/1, eLA/1
  Add19/1 -> Gain/1
  [HR] -> Gain3/1, Product15/2, Product15/1
  Gain2/1 -> Add18/1
  Constant20/1 -> Add19/2
  Product15/1 -> Gain2/1
  Gain3/1 -> Add18/2
  Add18/1 -> Add19/1

== system HMC/Reference CVSs/Pressures Flows and Volumes/Subsystem5/VolumesForVAD/Subsystem25 ==
  note: y = -0,1479x 2 + 38,021x - 923,75
  Add18 : Sum
  Add19 : Sum
  Constant20 : Constant  Value=-923.75
  Gain : Gain  Gain=1/10000
  Gain2 : Gain  Gain=-0.1479
  Gain3 : Gain  Gain=38.021
  Product15 : Product
  Scope : Scope
      settings: ActiveDisplayYMinimum=0.07241  ActiveDisplayYMaximum=0.09241
  eRA : Outport
  wires:
  Add19/1 -> Gain/1
  [HR] -> Gain3/1, Product15/2, Product15/1
  Constant20/1 -> Add19/2
  Add18/1 -> Add19/1
  Product15/1 -> Gain2/1
  Gain3/1 -> Add18/2
  Gain2/1 -> Add18/1
  Gain/1 -> Scope/1, eRA/1

== system HMC/Reference CVSs/Pressures Flows and Volumes/Subsystem5/VolumesForVAD/Subsystem26 ==
  note: y = -0,0225x 2 + 8,375x - 211,5
      | R² = 1
  note: y = 4,1667x2 + 3041,7x + 12500R² = 1
  Add18 : Sum
  Add19 : Sum
  Constant20 : Constant  Value=12500
  Gain : Gain  Gain=1/1000
  Gain2 : Gain  Gain=4.1667
  Gain3 : Gain  Gain=3041.7
  Product15 : Product
  Scope : Scope
      settings: ActiveDisplayYMinimum=197.50212  ActiveDisplayYMaximum=216.59303  DataLoggingVariableName=ScopeData2
  gLV : Outport
  wires:
  Gain/1 -> Scope/1, gLV/1
  Add18/1 -> Add19/1
  Gain3/1 -> Add18/2
  Product15/1 -> Gain2/1
  Constant20/1 -> Add19/2
  Gain2/1 -> Add18/1
  [HR] -> Product15/1, Product15/2, Gain3/1
  Add19/1 -> Gain/1

== system HMC/Reference CVSs/Pressures Flows and Volumes/Subsystem5/VolumesForVAD/Subsystem27 ==
  note: y = -0,0092x 2 + 3,2083x - 89,5
      | R² = 1
  note: y = 0,25x2 + 1212,5x - 3650R² = 1
  Add18 : Sum
  Add19 : Sum
  Constant20 : Constant  Value=-3650
  Gain : Gain  Gain=1/1000
  Gain2 : Gain  Gain=0.25
  Gain3 : Gain  Gain=1212.5
  Product15 : Product
  Scope : Scope
      settings: ActiveDisplayYMinimum=60  ActiveDisplayYMaximum=80  DataLoggingVariableName=ScopeData2
  gVt : Outport
  wires:
  Gain/1 -> Scope/1, gVt/1
  Add18/1 -> Add19/1
  Gain3/1 -> Add18/2
  Product15/1 -> Gain2/1
  Constant20/1 -> Add19/2
  Gain2/1 -> Add18/1
  [HR] -> Product15/1, Product15/2, Gain3/1
  Add19/1 -> Gain/1

== system HMC/Reference CVSs/Pressures Flows and Volumes/Subsystem5/VolumesForVAD/Subsystem28 ==
  note: y = -0,0208x 2 + 4,7917x - 162,5
  Add18 : Sum
  Add19 : Sum
  Constant20 : Constant  Value=-162.5
  Gain : Gain  Gain=1/10
  Gain2 : Gain  Gain=-0.0208
  Gain3 : Gain  Gain=4.7917
  Product15 : Product
  Scope : Scope
      settings: ActiveDisplayYMinimum=3.9997  ActiveDisplayYMaximum=5.9997  DataLoggingVariableName=ScopeData2
  gP : Outport
  wires:
  Gain/1 -> gP/1, Scope/1
  Add19/1 -> Gain/1
  [HR] -> Gain3/1, Product15/2, Product15/1
  Gain2/1 -> Add18/1
  Constant20/1 -> Add19/2
  Product15/1 -> Gain2/1
  Gain3/1 -> Add18/2
  Add18/1 -> Add19/1

== system HMC/Reference CVSs/Pressures Flows and Volumes/Subsystem5/VolumesForVAD/eAO resting1 ==
  note: y = 0,5x + 40
  Add19 : Sum
  Constant20 : Constant  Value=40
  Gain1 : Gain  Gain=1/100
  Gain3 : Gain  Gain=0.5
  Scope : Scope
      settings: ActiveDisplayYMinimum=0.50527  ActiveDisplayYMaximum=0.53249  DataLoggingVariableName=ScopeData2
  eAO : Outport
  wires:
  Gain1/1 -> Scope/1, eAO/1
  [insan] -> Gain3/1
  Constant20/1 -> Add19/2
  Gain3/1 -> Add19/1
  Add19/1 -> Gain1/1

== system HMC/Reference CVSs/Pressures Flows and Volumes/Subsystem5/VolumesForVAD/gao resting1 ==
  note: y = -0,0167x 2 + 3,25x - 45
  Add18 : Sum
  Add19 : Sum
  Constant20 : Constant  Value=-45
  Gain1 : Gain  Gain=1/100
  Gain2 : Gain  Gain=-0.0167
  Gain3 : Gain  Gain=3.25
  Product15 : Product
  Scope : Scope
      settings: ActiveDisplayYMinimum=0.88246  ActiveDisplayYMaximum=1.08246  DataLoggingVariableName=ScopeData2
  gAO : Outport
  wires:
  Add18/1 -> Add19/1
  Gain3/1 -> Add18/2
  Product15/1 -> Gain2/1
  Constant20/1 -> Add19/2
  Gain2/1 -> Add18/1
  [insan] -> Product15/1, Product15/2, Gain3/1
  Add19/1 -> Gain1/1
  Gain1/1 -> Scope/1, gAO/1

== system HMC/Reference CVSs/Pressures Flows and Volumes/Subsystem5/VolumesForVAD/hf10 ==
  note: y = 0,015x 2 - 2,25x + 301
  note: y = -2E-06x 2 + 0,0011x + 0,044
      | R² = 1
  note: y = -0,0069x2 + 1,2813x + 30,375R² = 1
  Add18 : Sum
  Add19 : Sum
  Constant20 : Constant  Value=301
  Gain : Gain  Gain=1/1000
  Gain2 : Gain  Gain=0.015
  Gain3 : Gain  Gain=-2.25
  Product15 : Product
  Scope : Scope
      settings: ActiveDisplayYMinimum=0.07241  ActiveDisplayYMaximum=0.09241
  eRA : Outport
  wires:
  Gain/1 -> eRA/1, Scope/1
  Gain2/1 -> Add18/1
  Gain3/1 -> Add18/2
  Product15/1 -> Gain2/1
  Add18/1 -> Add19/1
  Constant20/1 -> Add19/2
  [HR] -> Product15/1, Product15/2, Gain3/1
  Add19/1 -> Gain/1

== system HMC/Reference CVSs/Pressures Flows and Volumes/Subsystem5/VolumesForVAD/hf11 ==
  note: y = 0,0079x 2 - 0,7958x + 117,5
  note: y = -0,0073x2 + 26,677x - 591,88R² = 1
  note: y = -0,0014x 2 + 0,4834x - 14,119
      | R² = 1
  Add18 : Sum
  Add19 : Sum
  Constant20 : Constant  Value=117.5
  Gain1 : Gain  Gain=1/100
  Gain2 : Gain  Gain=0.0079
  Gain3 : Gain  Gain=-0.7958
  Product15 : Product
  Scope : Scope
      settings: ActiveDisplayYMinimum=0.88246  ActiveDisplayYMaximum=1.08246  DataLoggingVariableName=ScopeData2
  gAO : Outport
  wires:
  Add18/1 -> Add19/1
  Gain3/1 -> Add18/2
  Product15/1 -> Gain2/1
  Constant20/1 -> Add19/2
  Gain2/1 -> Add18/1
  [HR] -> Product15/1, Product15/2, Gain3/1
  Add19/1 -> Gain1/1
  Gain1/1 -> Scope/1, gAO/1

== system HMC/Reference CVSs/Pressures Flows and Volumes/Subsystem5/VolumesForVAD/hf12 ==
  note: y = 0,0222x 2 - 4,3333x + 230
  note: y = -0,1667x2 + 158,33x + 201100R² = 1
  note: y = -0,0008x 2 + 0,2917x + 195,5
      | R² = 1
  Add18 : Sum
  Add19 : Sum
  Constant20 : Constant  Value=230
  Gain2 : Gain  Gain=0.0222
  Gain3 : Gain  Gain=-4.3333
  Product15 : Product
  Scope : Scope
      settings: ActiveDisplayYMinimum=109.99968  ActiveDisplayYMaximum=309.99968  DataLoggingVariableName=ScopeData2
  gRV : Outport
  wires:
  [HR] -> Gain3/1, Product15/2, Product15/1
  Gain2/1 -> Add18/1
  Constant20/1 -> Add19/2
  Product15/1 -> Gain2/1
  Gain3/1 -> Add18/2
  Add18/1 -> Add19/1
  Add19/1 -> gRV/1, Scope/1

== system HMC/Reference CVSs/Pressures Flows and Volumes/Subsystem5/VolumesForVAD/hf7 ==
  note: y = 0,0167x 2 - 3,1667x + 240
  note: y = 0,0054x 2 - 1,6458x + 199,25
      | R² = 1
  Add18 : Sum
  Add19 : Sum
  Constant20 : Constant  Value=240
  Gain : Gain  Gain=1/1000
  Gain2 : Gain  Gain=0.0167
  Gain3 : Gain  Gain=-3.1667
  Product15 : Product
  Scope : Scope
      settings: ActiveDisplayYMinimum=0.01994  ActiveDisplayYMaximum=0.21994  DataLoggingVariableName=ScopeData2
  eP : Outport
  wires:
  Gain/1 -> Scope/1, eP/1
  Add18/1 -> Add19/1
  Gain3/1 -> Add18/2
  Product15/1 -> Gain2/1
  Constant20/1 -> Add19/2
  Gain2/1 -> Add18/1
  [HR] -> Product15/1, Product15/2, Gain3/1
  Add19/1 -> Gain/1

== system HMC/Reference CVSs/Pressures Flows and Volumes/Subsystem5/VolumesForVAD/hf8 ==
  note: y = -1E-16x 2 + 0,6667x - 3E-13
  Add18 : Sum
  Add19 : Sum
  Constant20 : Constant  Value=-3e-13
  Display : Display
  Gain1 : Gain  Gain=1/10000
  Gain2 : Gain  Gain=-1e-16
  Gain3 : Gain  Gain=0.6667
  Product15 : Product
  Scope : Scope
      settings: ActiveDisplayYMinimum=0.00132  ActiveDisplayYMaximum=0.00154  DataLoggingVariableName=ScopeData2
  eV : Outport
  wires:
  Add18/1 -> Add19/1
  Gain3/1 -> Add18/2
  Product15/1 -> Gain2/1
  Constant20/1 -> Add19/2
  Gain2/1 -> Add18/1
  [HR] -> Product15/1, Product15/2, Gain3/1
  Add19/1 -> Gain1/1
  Gain1/1 -> Scope/1, Display/1, eV/1

== system HMC/Reference CVSs/Pressures Flows and Volumes/Subsystem5/VolumesForVAD/hf9 ==
  note: y = -2E-06x 2 + 0,0011x + 0,044
      | R² = 1
  note: y = 0,0167x 2 - 2,8333x + 220
  Add18 : Sum
  Add19 : Sum
  Constant20 : Constant  Value=220
  Gain : Gain  Gain=1/1000
  Gain2 : Gain  Gain=0.0167
  Gain3 : Gain  Gain=-2.8333
  Product15 : Product
  Scope : Scope
      settings: ActiveDisplayYMinimum=0.07241  ActiveDisplayYMaximum=0.09241  DataLoggingVariableName=ScopeData2
  eLA : Outport
  wires:
  Add18/1 -> Add19/1
  Gain3/1 -> Add18/2
  Product15/1 -> Gain2/1
  Constant20/1 -> Add19/2
  Gain2/1 -> Add18/1
  [HR] -> Product15/1, Product15/2, Gain3/1
  Add19/1 -> Gain/1
  Gain/1 -> eLA/1, Scope/1

== system HMC/Reference CVSs/Pressures Flows and Volumes/Subsystem5/VolumesForVAD/hfao1 ==
  note: y = 3E-06x2 - 0,0008x + 0,5621R² = 1
  note: y = 0,0003x2 - 0,0823x + 56,212R² = 1
  note: y = 0,0271x2 - 8,2292x + 5621,2R² = 1
  Add18 : Sum
  Add19 : Sum
  Constant20 : Constant  Value=0.5621
  Gain2 : Gain  Gain=0.000003
  Gain3 : Gain  Gain=-0.0008
  Product15 : Product
  Scope : Scope
      settings: ActiveDisplayYMinimum=0.50527  ActiveDisplayYMaximum=0.53249  DataLoggingVariableName=ScopeData2
  eAO : Outport
  wires:
  [HR] -> Gain3/1, Product15/2, Product15/1
  Gain2/1 -> Add18/1
  Constant20/1 -> Add19/2
  Product15/1 -> Gain2/1
  Gain3/1 -> Add18/2
  Add18/1 -> Add19/1
  Add19/1 -> Scope/1, eAO/1
